simulink model "Pouziti_Expanze_moznosti"  (R2020b)
settings: Solver=VariableStepAuto  StartTime=0.0  StopTime=10.0  RelTol=1e-3  EnableMultiTasking=on
settings Model: Creator=Jirkovsk  LastModifiedBy=jirkovsky
settings DataIOCC: LimitDataPoints=on  SaveFormat=Array  SignalLoggingSaveFormat=ModelDataLogs  ReturnWorkspaceOutputs=off
settings OptimizationCC: ExpressionDepthLimit=2147483647  InitFltsAndDblsToZero=on  LifeSpan=inf
settings DebuggingCC: UnderspecifiedInitializationDetection=Classic  MergeDetectMultiDrivingBlocksExec=none  SolverPrmCheckMsg=warning  FcnCallInpInsideContextMsg=warning  StateNameClashWarn=warning  SFUnexpectedBacktrackingDiag=warning  SFNoUnconditionalDefaultTransitionDiag=warning  SFExecutionAtInitializationDiag=none  ArithmeticOperatorsInVariantConditions=warning
settings HardwareCC: ProdBitPerPointer=32  ProdBitPerSizeT=32  ProdBitPerPtrDiffT=32  ProdLargestAtomicFloat=None  ProdIntDivRoundTo=Undefined  ProdEndianess=Unspecified  ProdWordSize=32  ProdHWDeviceType=32-bit Generic
settings ModelReferenceCC: PropagateSignalLabelsOutOfModel=off
settings SFSimCC: SimUseLocalCustomCode=off  CustomCodeUndefinedFunction=UseInterfaceOnly
settings RTWCC: RTWUseLocalCustomCode=off
settings CodeAppCC: StateflowObjectComments=on
settings GRTTargetCC: TargetLangStandard=C89/C90 (ANSI)  CombineOutputUpdateFcns=off  GRTInterface=on
settings ConfigComp: CovMetricSettings=dw  CovSaveCumulativeToWorkspaceVar=on  CovSaveSingleToWorkspaceVar=on  CovExternalEMLEnable=off  CovSFcnEnable=off

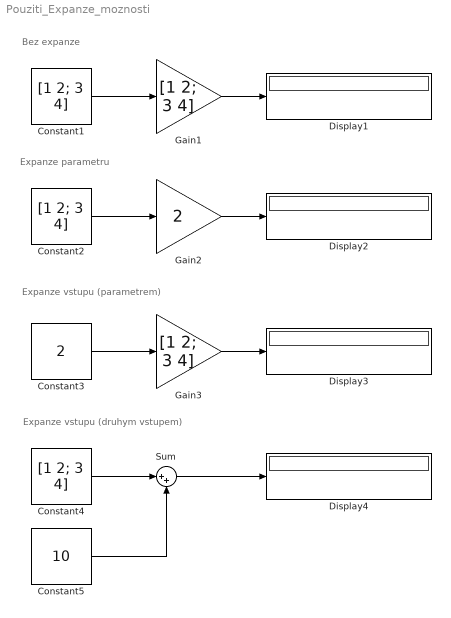
== system Pouziti_Expanze_moznosti ==
  note: Bez expanze
  note: Expanze parametru
  note: Expanze vstupu (parametrem)
  note: Expanze vstupu (druhym vstupem)
  Constant1 : Constant  Value=[1 2; 3 4]
  Constant2 : Constant  Value=[1 2; 3 4]
  Constant3 : Constant  Value=2
  Constant4 : Constant  Value=[1 2; 3 4]
  Constant5 : Constant  Value=10
  Display{1..4} (4 alike) : Display
  Gain1 : Gain  Gain=[1 2; 3 4]
  Gain2 : Gain  Gain=2
  Gain3 : Gain  Gain=[1 2; 3 4]
  Sum : Sum  Inputs=|++
  wires:
  Gain1/1 -> Display1/1
  Constant1/1 -> Gain1/1
  Gain2/1 -> Display2/1
  Constant2/1 -> Gain2/1
  Gain3/1 -> Display3/1
  Constant3/1 -> Gain3/1
  Sum/1 -> Display4/1
  Constant4/1 -> Sum/1
  Constant5/1 -> Sum/2
